simulink model "Tutorial_Simulink_6"  (R2024a)
settings: Solver=VariableStepAuto  StartTime=0.0  StopTime=10.0  MaxStep=.001  RelTol=1e-3
undefined symbols (not defined in the file): b, k, m
settings Model: Creator=gzipprich  LastModifiedBy=gzipprich

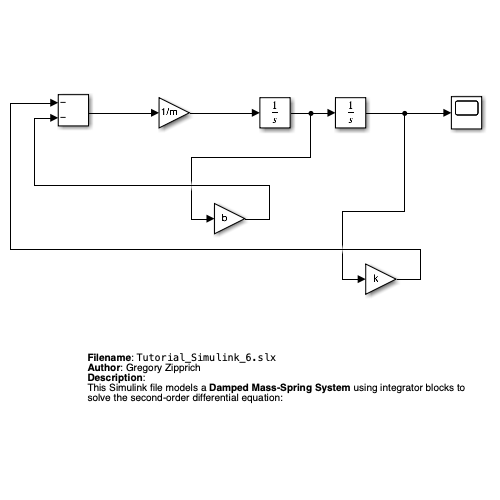
[thumbnail: Simulink's stored preview of the top-level diagram]
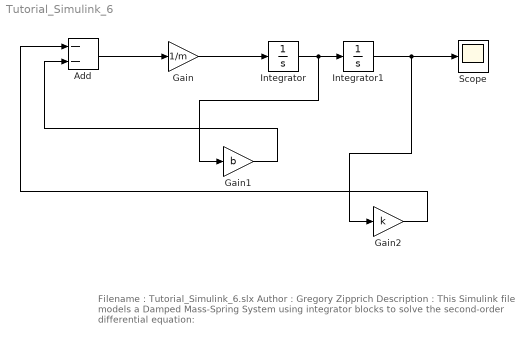
== system Tutorial_Simulink_6 ==
  note: Filename : Tutorial_Simulink_6.slx
      | Author : Gregory Zipprich
      | Description :
      | This Simulink file models a Damped Mass-Spring System using integrator blocks to solve the second-order differential equation:
  Add : Sum  Inputs=--
  Gain : Gain  Gain=1/m
  Gain1 : Gain  Gain=b
  Gain2 : Gain  Gain=k
  Integrator : Integrator
  Integrator1 : Integrator  InitialCondition=10
  Scope : Scope
  wires:
  Add/1 -> Gain/1
  Gain/1 -> Integrator/1
  Integrator/1 -> Gain1/1, Integrator1/1
  Integrator1/1 -> Gain2/1, Scope/1
  Gain1/1 -> Add/2
  Gain2/1 -> Add/1
